simulink model "motorPIcontrol"  (R2023a)
settings: Solver=FixedStepAuto  StartTime=0.0  StopTime=5  FixedStep=0.0001  RelTol=1e-3
settings Model: Creator=rout3  LastModifiedBy=rout3

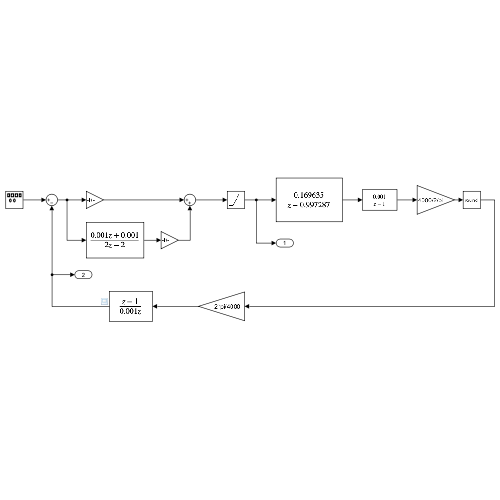
[thumbnail: Simulink's stored preview of the top-level diagram]
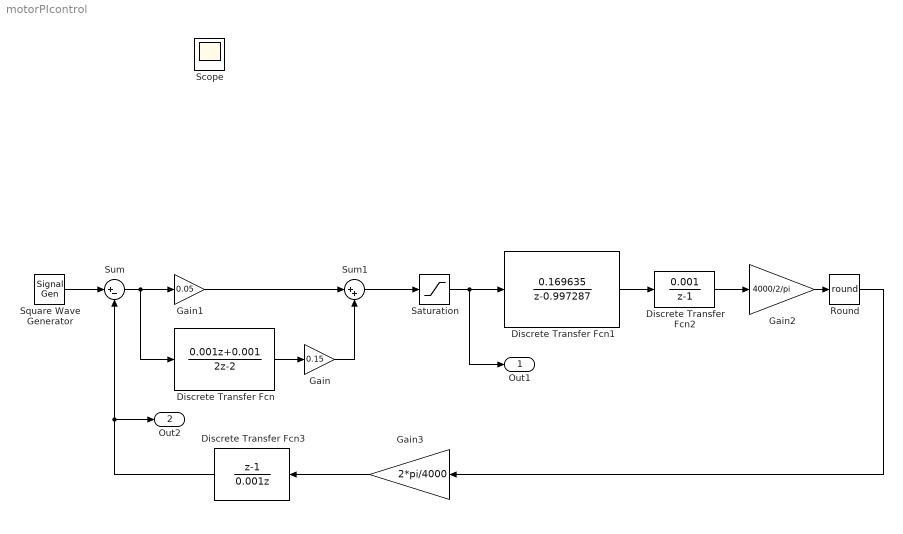
== system motorPIcontrol ==
  Discrete Transfer Fcn : DiscreteTransferFcn  Numerator=[0.001 0.001]  Denominator=[2 -2]  SampleTime=0.001
  Discrete Transfer Fcn1 : DiscreteTransferFcn  Numerator=[0.169635]  Denominator=[1 -0.997287]  SampleTime=0.001
  Discrete Transfer Fcn2 : DiscreteTransferFcn  Numerator=[0.001]  Denominator=[1 -1]  SampleTime=0.001
  Discrete Transfer Fcn3 : DiscreteTransferFcn  Numerator=[1 -1]  Denominator=[0.001 0]  SampleTime=0.001
  Gain : Gain  Gain=0.15
  Gain1 : Gain  Gain=0.05
  Gain2 : Gain  Gain=4000/2/pi
  Gain3 : Gain  Gain=2*pi/4000
  Round : Rounding  Operator=round
  Saturation : Saturate  UpperLimit=10  LowerLimit=-10
  Square Wave Generator : SignalGenerator  WaveForm=square  Amplitude=100  Frequency=0.25
  Sum : Sum  Inputs=|+-
  Sum1 : Sum  Inputs=|++
  Out1 : Outport
  Out2 : Outport  Port=2
  Scope : Scope
  wires:
  Discrete Transfer Fcn/1 -> Gain/1
  Sum/1 -> Discrete Transfer Fcn/1, Gain1/1
  Square Wave Generator/1 -> Sum/1
  Gain1/1 -> Sum1/1
  Gain/1 -> Sum1/2
  Sum1/1 -> Saturation/1
  Discrete Transfer Fcn1/1 -> Discrete Transfer Fcn2/1
  Gain2/1 -> Round/1
  Discrete Transfer Fcn2/1 -> Gain2/1
  Saturation/1 -> Out1/1, Discrete Transfer Fcn1/1
  Gain3/1 -> Discrete Transfer Fcn3/1
  Round/1 -> Gain3/1
  Discrete Transfer Fcn3/1 -> Sum/2, Out2/1
